simulink model "depthPhysics"  (R2016b)
settings: Solver=ode45  StartTime=0.0  StopTime=10.0  RelTol=1e-3  EnableMultiTasking=on
values from neighbouring files (symbols this model uses):
  Kd = rho*Cd*h*(lenZaxis/2)^3/3    (= 25)    [RSYawCTL_constants.m]
  rho = 1000    [RSYawCTL_constants.m]
undefined symbols (not defined in the file or in its folder): G, M, V
libraries: simulink x2
settings Model: Creator=Cassandra  LastModifiedBy=Cassandra
settings DataIOCC: LimitDataPoints=on  SaveFormat=Array
settings OptimizationCC: LifeSpan=inf
settings DebuggingCC: SFUnexpectedBacktrackingDiag=warning  SFNoUnconditionalDefaultTransitionDiag=warning  SFExecutionAtInitializationDiag=none
settings HardwareCC: ProdBitPerPointer=32  ProdBitPerSizeT=32  ProdBitPerPtrDiffT=32  ProdLargestAtomicFloat=None  ProdIntDivRoundTo=Undefined  ProdEndianess=Unspecified  ProdWordSize=32  ProdHWDeviceType=32-bit Generic
settings ModelReferenceCC: PropagateSignalLabelsOutOfModel=off
settings GRTTargetCC: TargetLangStandard=C89/C90 (ANSI)  GeneratePreprocessorConditionals=Disable all
settings ConfigComp: CovMetricSettings=dw  CovHtmlReporting=on  CovSaveCumulativeToWorkspaceVar=on  CovSaveSingleToWorkspaceVar=on  CovExternalEMLEnable=off

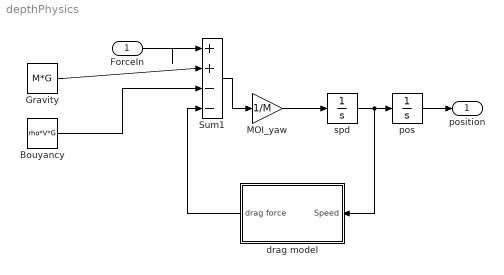
== system depthPhysics ==
  ForceIn : Inport
  Bouyancy : Constant  Value=rho*V*G
  Gravity : Constant  Value=M*G
  MOI_yaw : Gain  Gain=1/M
  Sum1 : Sum  Inputs=|++--
  drag model : Subsystem
  pos : Integrator
  spd : Integrator
  position : Outport
  wires:
  MOI_yaw/1 -> spd/1
  spd/1 -> pos/1, drag model/1(Speed)
  Sum1/1 -> MOI_yaw/1
  ForceIn/1 -> Sum1/1
  pos/1 -> position/1
  drag model/1(drag force) -> Sum1/4
  Gravity/1 -> Sum1/2
  Bouyancy/1 -> Sum1/3

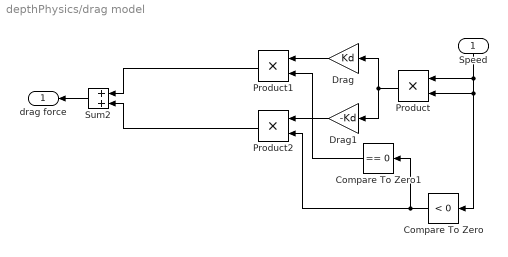
== system depthPhysics/drag model ==
  Speed : Inport
  Compare To Zero : simulink/Logic and Bit Operations/Compare To Zero  relop=<  OutDataTypeStr=boolean
  Compare To Zero1 : simulink/Logic and Bit Operations/Compare To Zero  relop===  OutDataTypeStr=boolean
  Drag : Gain  Gain=Kd
  Drag1 : Gain  Gain=-Kd
  Product : Product
  Product1 : Product
  Product2 : Product
  Sum2 : Sum  Inputs=+|+
  drag force : Outport
  wires:
  Speed/1 -> Product/1, Compare To Zero/1, Product/2
  Drag1/1 -> Product2/1
  Compare To Zero1/1 -> Product1/2
  Product1/1 -> Sum2/1
  Drag/1 -> Product1/1
  Sum2/1 -> drag force/1
  Product/1 -> Drag1/1, Drag/1
  Product2/1 -> Sum2/2
  Compare To Zero/1 -> Product2/2, Compare To Zero1/1
